simulink model "mavsim_modify"  (R2018b)
settings: Solver=ode15s  StartTime=0.0  StopTime=200  FixedStep=P.Ts  RelTol=1e-3  EnableMultiTasking=on
InitFcn:
  | aerosonde
  | param_chap7
values from neighbouring files (symbols this model uses):
  q = uu(11)    [drawVehicle.m]    (also in forceee.m; plotmavstatevariables.m = 180/pi*uu(11); plotresults.m = 180/pi*uu(11))
  r = uu(12)    [drawVehicle.m]    (also in forceee.m; plotmavstatevariables.m = 180/pi*uu(12); plotresults.m = 180/pi*uu(12))
undefined symbols (not defined in the file or in its folder): altitude_state_machine, drawVehicle, forceee, forces_moments, gps, HDBK, Light, MIL, P, plotmavstatevariables, plotresults, sensors, true_states
libraries: aerolibwind2 x2, simulink x2, simulink_extras x1, aerolibobsolete x1
settings Model: Creator=beard  LastModifiedBy=xinyizhao
settings DataIOCC: LimitDataPoints=on  SaveFormat=Array  SignalLoggingSaveFormat=ModelDataLogs
settings OptimizationCC: ExpressionDepthLimit=2147483647  InitFltsAndDblsToZero=on  LifeSpan=inf
settings DebuggingCC: UnderspecifiedInitializationDetection=Classic  MergeDetectMultiDrivingBlocksExec=none  SolverPrmCheckMsg=warning  FcnCallInpInsideContextMsg=warning  StateNameClashWarn=warning  LibraryContextMissingDiagnostic=none  SFUnexpectedBacktrackingDiag=warning  SFNoUnconditionalDefaultTransitionDiag=warning  SFExecutionAtInitializationDiag=none
settings HardwareCC: ProdBitPerPointer=32  ProdBitPerSizeT=32  ProdBitPerPtrDiffT=32  ProdLargestAtomicFloat=None  ProdIntDivRoundTo=Undefined  ProdEndianess=Unspecified  ProdWordSize=32  ProdHWDeviceType=32-bit Generic
settings ModelReferenceCC: PropagateSignalLabelsOutOfModel=off
settings SFSimCC: SimUseLocalCustomCode=off
settings RTWCC: RTWUseLocalCustomCode=off
settings CodeAppCC: StateflowObjectComments=on
settings GRTTargetCC: TargetLangStandard=C89/C90 (ANSI)  GeneratePreprocessorConditionals=Disable all  CombineOutputUpdateFcns=off  GRTInterface=on
settings ConfigComp: CovMetricSettings=dw  CovHtmlReporting=on  CovSaveCumulativeToWorkspaceVar=on  CovSaveSingleToWorkspaceVar=on  CovExternalEMLEnable=off  CovSFcnEnable=off

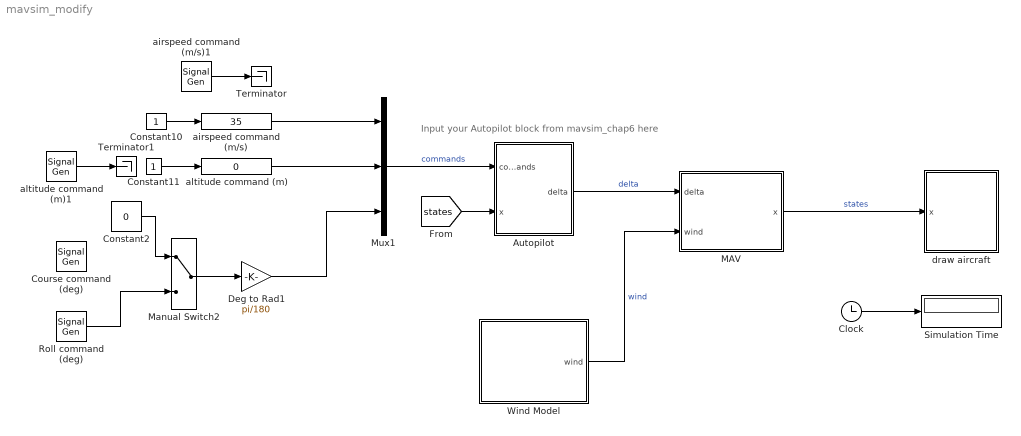
== system mavsim_modify ==
  note: Input your Autopilot block from mavsim_chap6 here
  Autopilot : Subsystem
      mask Display: image(imread('px4.png'))
  Clock : Clock
  Constant10 : Constant
  Constant11 : Constant
  Constant2 : Constant  Value=0
  Course command (deg) : SignalGenerator  WaveForm=square  Amplitude=20  Frequency=.05
  Deg to Rad1 : Gain  Gain=pi/180
  MAV : Subsystem
      mask Display: image(imread('mav.png'))
  Manual Switch2 : ManualSwitch
  Mux1 : Mux  Inputs=3
  Roll command (deg) : SignalGenerator  WaveForm=square  Amplitude=20  Frequency=.05
  Simulation Time : Display
  Terminator : Terminator
  Terminator1 : Terminator
  Wind Model : Subsystem
      mask Display: image('wind.jpg');
  airspeed command (m/s) : simulink/Math Operations/Slider Gain  gain=35  low=5  high=50
  airspeed command (m/s)1 : SignalGenerator  WaveForm=square  Amplitude=4  Frequency=.02
  altitude command (m) : simulink/Math Operations/Slider Gain  gain=0  low=0  high=500
  altitude command (m)1 : SignalGenerator  WaveForm=square  Amplitude=20  Frequency=.03
  draw aircraft : Subsystem
      mask Display: image(imread('tv.jpg'))
  wires:
  Clock/1 -> Simulation Time/1
  Wind Model/1(wind) -> MAV/2(wind)  "wind"
  MAV/1(x) -> draw aircraft/1(x)  "states"
  Autopilot/1(delta) -> MAV/1(delta)  "delta"
  Mux1/1 -> Autopilot/1(commands)  "commands"
  [states] -> Autopilot/2(x)
  Constant10/1 -> airspeed command (m/s)/1
  Deg to Rad1/1 -> Mux1/3
  airspeed command (m/s)/1 -> Mux1/1
  Constant11/1 -> altitude command (m)/1
  altitude command (m)/1 -> Mux1/2
  Manual Switch2/1 -> Deg to Rad1/1
  Roll command (deg)/1 -> Manual Switch2/2
  Constant2/1 -> Manual Switch2/1
  airspeed command (m/s)1/1 -> Terminator/1
  altitude command (m)1/1 -> Terminator1/1

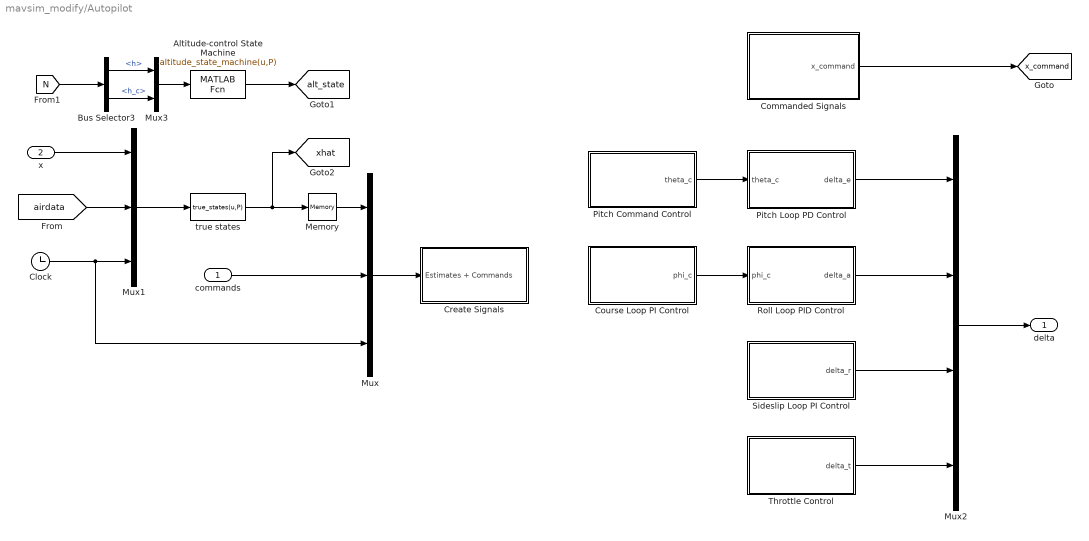
== system mavsim_modify/Autopilot ==
  commands : Inport
  x : Inport  Port=2
  Altitude-control State Machine : MATLABFcn  MATLABFcn=altitude_state_machine(u,P)  OutputDimensions=1  SampleTime=P.Ts
  Bus Selector3 : BusSelector  OutputSignals=h,h_c
  Clock : Clock
  Commanded Signals : Subsystem
  Course Loop PI Control : Subsystem
  Create Signals : Subsystem
  Memory : Memory
  Mux : Mux  Inputs=3
  Mux1 : Mux  Inputs=3
  Mux2 : Mux
  Mux3 : Mux  Inputs=2
  Pitch Command Control : Subsystem
  Pitch Loop PD Control : Subsystem
  Roll Loop PID Control : Subsystem
  Sideslip Loop PI Control : Subsystem
  Throttle Control : Subsystem
  true states : MATLABFcn  MATLABFcn=true_states(u,P)  OutputDimensions=19  SampleTime=P.Ts
  delta : Outport
  tag scope: alt_state=global, x_command=global, xhat=global
  wires:
  Clock/1 -> Mux/3, Mux1/3
  Mux2/1 -> delta/1
  commands/1 -> Mux/2
  Mux1/1 -> true states/1
  x/1 -> Mux1/1
  true states/1 -> [xhat], Memory/1
  [airdata] -> Mux1/2
  Memory/1 -> Mux/1
  Mux/1 -> Create Signals/1(Estimates + Commands)
  Pitch Loop PD Control/1(delta_e) -> Mux2/1
  Sideslip Loop PI Control/1(delta_r) -> Mux2/3
  Throttle Control/1(delta_t) -> Mux2/4
  Commanded Signals/1(x_command) -> [x_command]
  Altitude-control State Machine/1 -> [alt_state]
  [N] -> Bus Selector3/1
  Bus Selector3/1 -> Mux3/1  "<h>"
  Pitch Command Control/1(theta_c) -> Pitch Loop PD Control/1(theta_c)
  Bus Selector3/2 -> Mux3/2  "<h_c>"
  Mux3/1 -> Altitude-control State Machine/1
  Course Loop PI Control/1(phi_c) -> Roll Loop PID Control/1(phi_c)
  Roll Loop PID Control/1(delta_a) -> Mux2/2

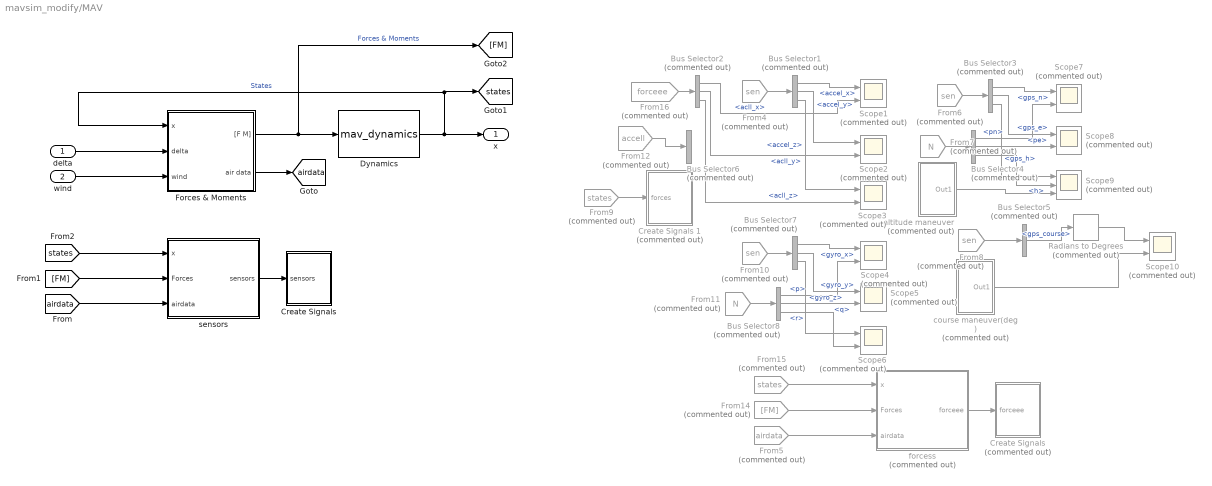
== system mavsim_modify/MAV ==
  delta : Inport
  wind : Inport  Port=2
  Bus Selector1 : BusSelector  Commented=on  OutputSignals=accel_x,accel_y,accel_z
  Bus Selector2 : BusSelector  Commented=on  OutputSignals=acll_x,acll_y,acll_z
  Bus Selector3 : BusSelector  Commented=on  OutputSignals=gps_n,gps_e,gps_h
  Bus Selector4 : BusSelector  Commented=on  OutputSignals=pn,pe,h
  Bus Selector5 : BusSelector  Commented=on  OutputSignals=gps_course
  Bus Selector6 : BusSelector  Commented=on  OutputSignals=u_dot,v_dot,w_dot
  Bus Selector7 : BusSelector  Commented=on  OutputSignals=gyro_x,gyro_y,gyro_z
  Bus Selector8 : BusSelector  Commented=on  OutputSignals=p,q,r
  Create Signals : Subsystem
  "Create Signals " : Subsystem  Commented=on
  Create Signals 1 : Subsystem  Commented=on
  Dynamics : S-Function  FunctionName=mav_dynamics  Parameters=P  SFunctionDeploymentMode=off  EnableBusSupport=off
  Forces & Moments : Subsystem
  From{4,6,8,10} (4 alike) : From  Commented=on  GotoTag=sen  TagVisibility=global
  From11 : From  Commented=on  GotoTag=N  TagVisibility=global
  From12 : From  Commented=on  GotoTag=accell  TagVisibility=global
  From14 : From  Commented=on  GotoTag=FM
  From15 : From  Commented=on  GotoTag=states  TagVisibility=global
  From16 : From  Commented=on  GotoTag=forceee  TagVisibility=global
  From5 : From  Commented=on  GotoTag=airdata  TagVisibility=global
  From7 : From  Commented=on  GotoTag=N  TagVisibility=global
  From9 : From  Commented=on  GotoTag=states  TagVisibility=global
  Radians to Degrees : simulink_extras/Transformations/Radians to Degrees  Commented=on
  Scope{1..8,10} (9 alike) : Scope  Commented=on  NumInputPorts=2
  Scope9 : Scope  Commented=on  NumInputPorts=3
  altitude maneuver : Subsystem  Commented=on
  course maneuver(deg) : Subsystem  Commented=on
  forcess : Subsystem  Commented=on
  sensors : Subsystem
  x : Outport
  tag scope: airdata=global, states=global
  wires:
  Dynamics/1 -> [states], Forces & Moments/1(x), x/1  "States"
  Forces & Moments/1("[F M]") -> [FM], Dynamics/1  "Forces & Moments"
  Forces & Moments/2(air data) -> [airdata]
  delta/1 -> Forces & Moments/2(delta)
  wind/1 -> Forces & Moments/3(wind)
  [airdata] -> sensors/3(airdata)
  [FM] -> sensors/2(Forces)
  [states] -> sensors/1(x)
  sensors/1(sensors) -> Create Signals/1(sensors)
  Bus Selector1/3 -> Scope3/1  "<accel_z>"
  From11/1 -> Bus Selector8/1
  From10/1 -> Bus Selector7/1
  Bus Selector7/2 -> Scope5/1  "<gyro_y>"
  From4/1 -> Bus Selector1/1
  Radians to Degrees/1 -> Scope10/1
  Bus Selector4/3 -> Scope9/2  "<h>"
  Bus Selector5/1 -> Radians to Degrees/1  "<gps_course>"
  From6/1 -> Bus Selector3/1
  Bus Selector7/1 -> Scope4/1  "<gyro_x>"
  Bus Selector8/1 -> Scope4/2  "<p>"
  Bus Selector1/1 -> Scope1/1  "<accel_x>"
  Bus Selector1/2 -> Scope2/1  "<accel_y>"
  Bus Selector3/2 -> Scope8/1  "<gps_e>"
  Bus Selector4/1 -> Scope7/2  "<pn>"
  Bus Selector8/2 -> Scope5/2  "<q>"
  Bus Selector3/3 -> Scope9/1  "<gps_h>"
  Bus Selector8/3 -> Scope6/2  "<r>"
  Bus Selector7/3 -> Scope6/1  "<gyro_z>"
  Bus Selector4/2 -> Scope8/2  "<pe>"
  Bus Selector3/1 -> Scope7/1  "<gps_n>"
  From7/1 -> Bus Selector4/1
  course maneuver(deg)/1(Out1) -> Scope10/2
  From8/1 -> Bus Selector5/1
  From5/1 -> forcess/3(airdata)
  forcess/1(forceee) -> "Create Signals "/1(forceee)
  From15/1 -> forcess/1(x)
  From14/1 -> forcess/2(Forces)
  From16/1 -> Bus Selector2/1
  From9/1 -> Create Signals 1/1(forces)
  From12/1 -> Bus Selector6/1
  Bus Selector2/1 -> Scope1/2  "<acll_x>"
  Bus Selector2/2 -> Scope2/2  "<acll_y>"
  Bus Selector2/3 -> Scope3/2  "<acll_z>"
  altitude maneuver/1(Out1) -> Scope9/3

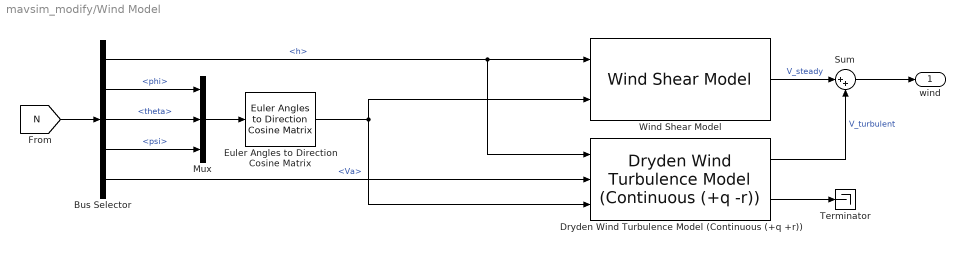
== system mavsim_modify/Wind Model ==
  Bus Selector : BusSelector  OutputSignals=h,phi,theta,psi,Va
  Dryden Wind Turbulence Model (Continuous (+q +r)) : aerolibwind2/Dryden Wind Turbulence Model  (Continuous (+q -r))  units=Metric (MKS)  spec=MIL-HDBK-1797  model=Continuous Dryden (+q +r)  W20=P.w_mag  Wdeg=P.w_dir  TurbProb=10^-2 - Light  L_high=533.4  Wingspan=P.b  ts=P.Ts  Seed=[23341 23342 0 23344]  T_on=off
      settings: SourceProductName=Aerospace Blockset
  Euler Angles to Direction Cosine Matrix : aerolibobsolete/Euler Angles to  Direction Cosine Matrix
      settings: SourceProductName=Aerospace Blockset  SourceProductBaseCode=AE
  Mux : Mux  Inputs=3
  Sum : Sum  Inputs=|++
  Terminator : Terminator
  Wind Shear Model : aerolibwind2/Wind Shear Model  units=Metric (MKS)  phase=Category C - Terminal Flight Phase  W_20=P.w_mag  Wdeg=P.w_dir
      settings: SourceProductName=Aerospace Blockset
  wind : Outport
  wires:
  Dryden Wind Turbulence Model (Continuous (+q +r))/2 -> Terminator/1
  Euler Angles to Direction Cosine Matrix/1 -> Dryden Wind Turbulence Model (Continuous (+q +r))/3, Wind Shear Model/2
  Wind Shear Model/1 -> Sum/1  "V_steady"
  Bus Selector/5 -> Dryden Wind Turbulence Model (Continuous (+q +r))/2  "<Va>"
  Bus Selector/1 -> Dryden Wind Turbulence Model (Continuous (+q +r))/1, Wind Shear Model/1  "<h>"
  Dryden Wind Turbulence Model (Continuous (+q +r))/1 -> Sum/2  "V_turbulent"
  Bus Selector/2 -> Mux/1  "<phi>"
  Bus Selector/3 -> Mux/2  "<theta>"
  Bus Selector/4 -> Mux/3  "<psi>"
  Mux/1 -> Euler Angles to Direction Cosine Matrix/1
  Sum/1 -> wind/1
  [N] -> Bus Selector/1

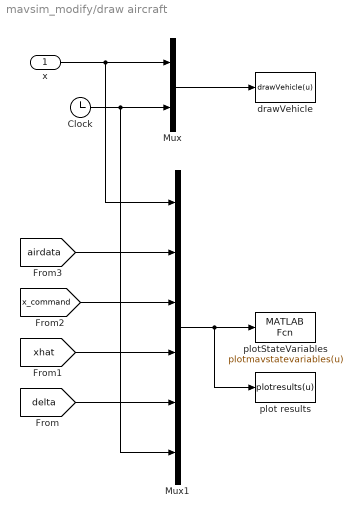
== system mavsim_modify/draw aircraft ==
  x : Inport
  Clock : Clock
  Mux : Mux  Inputs=2
  Mux1 : Mux  Inputs=6
  drawVehicle : MATLABFcn  MATLABFcn=drawVehicle(u)  OutputDimensions=0  SampleTime=0.1
  plot results : MATLABFcn  MATLABFcn=plotresults(u)  OutputDimensions=0  SampleTime=0.1
  plotStateVariables : MATLABFcn  MATLABFcn=plotmavstatevariables(u)  OutputDimensions=0  SampleTime=0.1
  wires:
  Mux/1 -> drawVehicle/1
  x/1 -> Mux/1, Mux1/1
  Clock/1 -> Mux/2, Mux1/6
  [xhat] -> Mux1/4
  [x_command] -> Mux1/3
  [delta] -> Mux1/5
  [airdata] -> Mux1/2
  Mux1/1 -> plot results/1, plotStateVariables/1

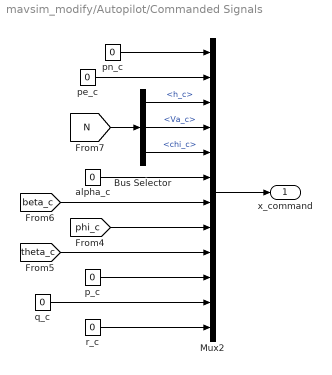
== system mavsim_modify/Autopilot/Commanded Signals ==
  Bus Selector : BusSelector  OutputSignals=h_c,Va_c,chi_c
  Mux2 : Mux  Inputs=12
  alpha_c : Constant  Value=0
  p_c : Constant  Value=0
  pe_c : Constant  Value=0
  pn_c : Constant  Value=0
  q_c : Constant  Value=0
  r_c : Constant  Value=0
  x_command : Outport
  wires:
  Bus Selector/1 -> Mux2/3  "<h_c>"
  pe_c/1 -> Mux2/2
  p_c/1 -> Mux2/10
  Mux2/1 -> x_command/1
  alpha_c/1 -> Mux2/6
  pn_c/1 -> Mux2/1
  Bus Selector/2 -> Mux2/4  "<Va_c>"
  [beta_c] -> Mux2/7
  Bus Selector/3 -> Mux2/5  "<chi_c>"
  q_c/1 -> Mux2/11
  [N] -> Bus Selector/1
  r_c/1 -> Mux2/12
  [phi_c] -> Mux2/8
  [theta_c] -> Mux2/9

== system mavsim_modify/Autopilot/Course Loop PI Control ==
  Bus Selector3 : BusSelector  OutputSignals=chi_c,chi
  Gain : Gain  Gain=P.course_kp
  Roll Saturation : Saturate  UpperLimit=P.phi_max  LowerLimit=-1*P.phi_max
  Sum : Sum
  Sum4 : Sum  Inputs=|+-
  course_ki : TransferFcn  Numerator=[P.course_ki]  Denominator=[1 0]
  phi_c : Outport
  wires:
  [N] -> Bus Selector3/1
  Bus Selector3/2 -> Sum4/2  "<chi>"
  Bus Selector3/1 -> Sum4/1  "<chi_c>"
  Roll Saturation/1 -> phi_c/1
  Sum4/1 -> Gain/1, course_ki/1  "course_e"
  Gain/1 -> Sum/2
  course_ki/1 -> Sum/1
  Sum/1 -> Roll Saturation/1

== system mavsim_modify/Autopilot/Create Signals ==
  Estimates + Commands : Inport
  Bus Creator : BusCreator  Inputs=23
  Demux1 : Demux  Outputs=23
  tag scope: N=global
  wires:
  Demux1/14 -> Bus Creator/14  "wn"
  Demux1/4 -> Bus Creator/4  "Va"
  Demux1/2 -> Bus Creator/2  "pe"
  Demux1/21 -> Bus Creator/21  "h_c"
  Demux1/15 -> Bus Creator/15  "we"
  Demux1/13 -> Bus Creator/13  "Vg"
  Demux1/18 -> Bus Creator/18  "by"
  Estimates + Commands/1 -> Demux1/1
  Demux1/9 -> Bus Creator/9  "chi"
  Demux1/17 -> Bus Creator/17  "bx"
  Demux1/16 -> Bus Creator/16  "psi"
  Demux1/20 -> Bus Creator/20  "Va_c"
  Demux1/19 -> Bus Creator/19  "bz"
  Demux1/5 -> Bus Creator/5  "alpha"
  Demux1/23 -> Bus Creator/23  "t"
  Demux1/10 -> Bus Creator/10  "p"
  Demux1/12 -> Bus Creator/12  "r"
  Demux1/11 -> Bus Creator/11  "q"
  Bus Creator/1 -> [N]
  Demux1/22 -> Bus Creator/22  "chi_c"
  Demux1/3 -> Bus Creator/3  "h"
  Demux1/8 -> Bus Creator/8  "theta"
  Demux1/6 -> Bus Creator/6  "beta"
  Demux1/7 -> Bus Creator/7  "phi"
  Demux1/1 -> Bus Creator/1  "pn"

== system mavsim_modify/Autopilot/Pitch Command Control ==
  Airspeed Hold Using Pitch Loop PI Control : Subsystem
  "Airspeed Hold Using Pitch Loop PI Control " : Subsystem
  Altitude Hold Using Pitch Loop PI Control : Subsystem
  Constant : Constant  Value=P.theta_max
  Multiport Switch : MultiPortSwitch  Inputs=4  DataPortIndices={10,2,3}  DiagnosticForDefault=None
  Pitch Saturation : Saturate  UpperLimit=P.theta_max  LowerLimit=-1*P.theta_max
  theta_c : Outport
  wires:
  Altitude Hold Using Pitch Loop PI Control/1(theta_c) -> Multiport Switch/4  "Altitude Hold Zone"
  Airspeed Hold Using Pitch Loop PI Control/1(theta_c) -> Multiport Switch/3  "Climb Zone"
  [alt_state] -> Multiport Switch/1  "Altitude-control State Variable"
  Constant/1 -> Multiport Switch/2  "Take-off Zone"
  "Airspeed Hold Using Pitch Loop PI Control "/1(theta_c) -> Multiport Switch/5  "Descend Zone"
  Multiport Switch/1 -> Pitch Saturation/1
  Pitch Saturation/1 -> theta_c/1

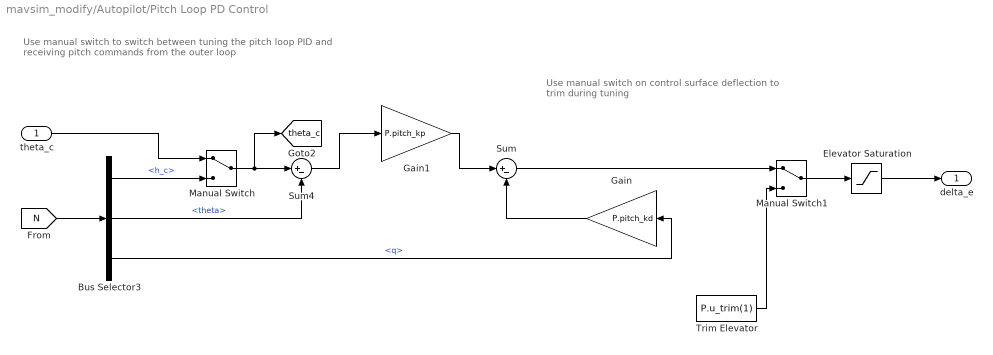
== system mavsim_modify/Autopilot/Pitch Loop PD Control ==
  note: Use manual switch to switch between tuning the pitch loop PID and
      | receiving pitch commands from the outer loop
  note: Use manual switch on control surface deflection
      | to trim during tuning
  theta_c : Inport
  Bus Selector3 : BusSelector  OutputSignals=h_c,theta,q
  Elevator Saturation : Saturate  UpperLimit=P.delta_e_max  LowerLimit=-1*P.delta_e_max
  Gain : Gain  Gain=P.pitch_kd
  Gain1 : Gain  Gain=P.pitch_kp
  Manual Switch : ManualSwitch
  Manual Switch1 : ManualSwitch
  Sum : Sum  Inputs=|+-
  Sum4 : Sum  Inputs=|+-
  Trim Elevator : Constant  Value=P.u_trim(1)
  delta_e : Outport
  tag scope: theta_c=global
  wires:
  Manual Switch/1 -> [theta_c], Sum4/1
  theta_c/1 -> Manual Switch/1
  [N] -> Bus Selector3/1
  Bus Selector3/2 -> Sum4/2  "<theta>"
  Bus Selector3/1 -> Manual Switch/2  "<h_c>"
  Trim Elevator/1 -> Manual Switch1/2
  Manual Switch1/1 -> Elevator Saturation/1
  Sum4/1 -> Gain1/1
  Bus Selector3/3 -> Gain/1  "<q>"
  Gain1/1 -> Sum/1
  Gain/1 -> Sum/2
  Sum/1 -> Manual Switch1/1
  Elevator Saturation/1 -> delta_e/1

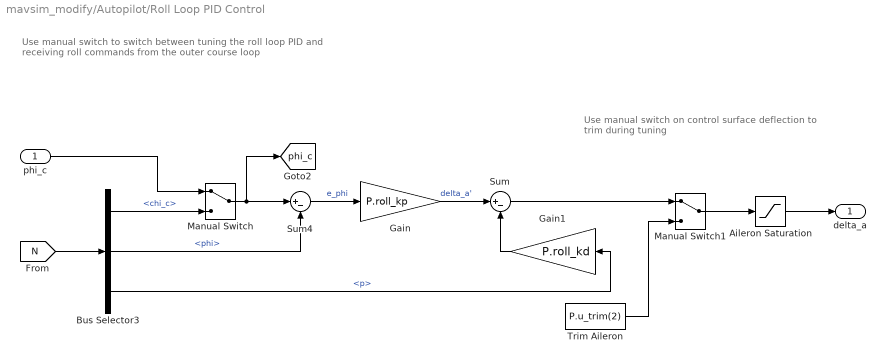
== system mavsim_modify/Autopilot/Roll Loop PID Control ==
  note: Use manual switch on control surface deflection
      | to trim during tuning
  note: Use manual switch to switch between tuning the roll loop PID and
      | receiving roll commands from the outer course loop
  phi_c : Inport
  Aileron Saturation : Saturate  UpperLimit=P.delta_a_max  LowerLimit=-1*P.delta_a_max
  Bus Selector3 : BusSelector  OutputSignals=chi_c,phi,p
  Gain : Gain  Gain=P.roll_kp
  Gain1 : Gain  Gain=P.roll_kd
  Manual Switch : ManualSwitch
  Manual Switch1 : ManualSwitch
  Sum : Sum  Inputs=|+-
  Sum4 : Sum  Inputs=|+-
  Trim Aileron : Constant  Value=P.u_trim(2)
  delta_a : Outport
  tag scope: phi_c=global
  wires:
  Bus Selector3/1 -> Manual Switch/2  "<chi_c>"
  Bus Selector3/2 -> Sum4/2  "<phi>"
  [N] -> Bus Selector3/1
  phi_c/1 -> Manual Switch/1
  Manual Switch/1 -> [phi_c], Sum4/1
  Aileron Saturation/1 -> delta_a/1
  Trim Aileron/1 -> Manual Switch1/2
  Manual Switch1/1 -> Aileron Saturation/1
  Sum4/1 -> Gain/1  "e_phi"
  Gain/1 -> Sum/1  "delta_a'"
  Gain1/1 -> Sum/2
  Sum/1 -> Manual Switch1/1
  Bus Selector3/3 -> Gain1/1  "<p>"

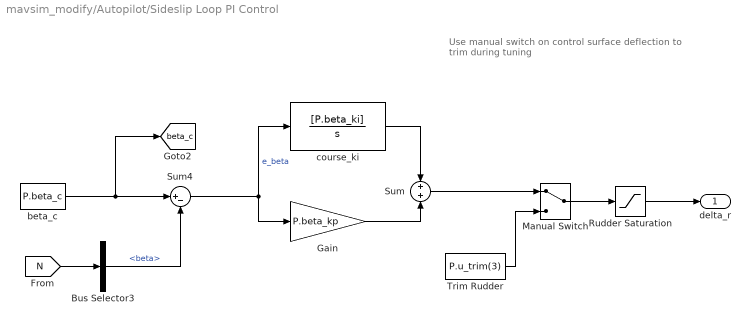
== system mavsim_modify/Autopilot/Sideslip Loop PI Control ==
  note: Use manual switch on control surface deflection
      | to trim during tuning
  Bus Selector3 : BusSelector  OutputSignals=beta
  Gain : Gain  Gain=P.beta_kp
  Manual Switch : ManualSwitch
  Rudder Saturation : Saturate  UpperLimit=P.delta_r_max  LowerLimit=-1*P.delta_r_max
  Sum : Sum
  Sum4 : Sum  Inputs=|+-
  Trim Rudder : Constant  Value=P.u_trim(3)
  beta_c : Constant  Value=P.beta_c
  course_ki : TransferFcn  Numerator=[P.beta_ki]  Denominator=[1 0]
  delta_r : Outport
  tag scope: beta_c=global
  wires:
  [N] -> Bus Selector3/1
  Bus Selector3/1 -> Sum4/2  "<beta>"
  beta_c/1 -> [beta_c], Sum4/1
  Manual Switch/1 -> Rudder Saturation/1
  Trim Rudder/1 -> Manual Switch/2
  Rudder Saturation/1 -> delta_r/1
  Sum4/1 -> Gain/1, course_ki/1  "e_beta"
  course_ki/1 -> Sum/1
  Sum/1 -> Manual Switch/1
  Gain/1 -> Sum/2

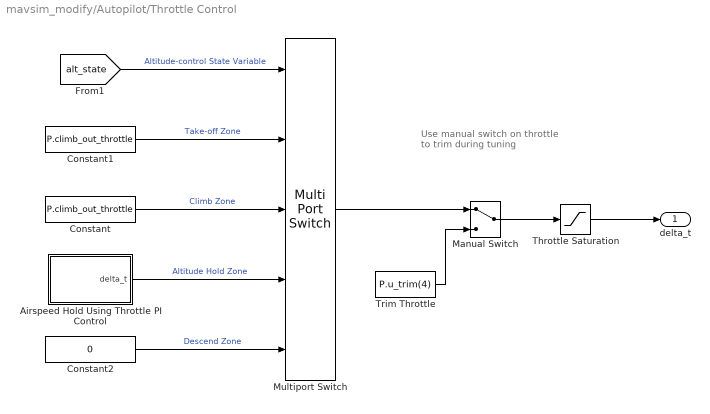
== system mavsim_modify/Autopilot/Throttle Control ==
  note: Use manual switch on throttle
      | to trim during tuning
  Airspeed Hold Using Throttle PI Control : Subsystem
  Constant : Constant  Value=P.climb_out_throttle
  Constant1 : Constant  Value=P.climb_out_throttle
  Constant2 : Constant  Value=0
  Manual Switch : ManualSwitch
  Multiport Switch : MultiPortSwitch  Inputs=4  DataPortIndices={10,2,3}  DiagnosticForDefault=None
  Throttle Saturation : Saturate  UpperLimit=P.throttle_max  LowerLimit=0
  Trim Throttle : Constant  Value=P.u_trim(4)
  delta_t : Outport
  wires:
  Multiport Switch/1 -> Manual Switch/1
  Airspeed Hold Using Throttle PI Control/1(delta_t) -> Multiport Switch/4  "Altitude Hold Zone"
  [alt_state] -> Multiport Switch/1  "Altitude-control State Variable"
  Constant/1 -> Multiport Switch/3  "Climb Zone"
  Constant1/1 -> Multiport Switch/2  "Take-off Zone"
  Constant2/1 -> Multiport Switch/5  "Descend Zone"
  Throttle Saturation/1 -> delta_t/1
  Trim Throttle/1 -> Manual Switch/2
  Manual Switch/1 -> Throttle Saturation/1

== system mavsim_modify/MAV/Create Signals ==
  sensors : Inport
  Bus Creator : BusCreator  Inputs=13
  Demux1 : Demux  Outputs=13
  tag scope: sen=global
  wires:
  sensors/1 -> Demux1/1
  Bus Creator/1 -> [sen]
  Demux1/1 -> Bus Creator/1  "gyro_x"
  Demux1/2 -> Bus Creator/2  "gyro_y"
  Demux1/3 -> Bus Creator/3  "gyro_z"
  Demux1/4 -> Bus Creator/4  "accel_x"
  Demux1/5 -> Bus Creator/5  "accel_y"
  Demux1/6 -> Bus Creator/6  "accel_z"
  Demux1/7 -> Bus Creator/7  "static_pres"
  Demux1/8 -> Bus Creator/8  "diff_pres"
  Demux1/9 -> Bus Creator/9  "gps_n"
  Demux1/10 -> Bus Creator/10  "gps_e"
  Demux1/11 -> Bus Creator/11  "gps_h"
  Demux1/12 -> Bus Creator/12  "gps_Vg"
  Demux1/13 -> Bus Creator/13  "gps_course"

== system mavsim_modify/MAV/Create Signals  ==
  forceee : Inport
  Bus Creator : BusCreator  Inputs=3
  Demux1 : Demux  Outputs=3
  tag scope: forceee=global
  wires:
  forceee/1 -> Demux1/1
  Bus Creator/1 -> [forceee]
  Demux1/1 -> Bus Creator/1  "acll_x"
  Demux1/2 -> Bus Creator/2  "acll_y"
  Demux1/3 -> Bus Creator/3  "acll_z"

== system mavsim_modify/MAV/Create Signals 1 ==
  forces : Inport
  Bus Creator : BusCreator  Inputs=12
  Demux1 : Demux  Outputs=12
  tag scope: accell=global
  wires:
  forces/1 -> Demux1/1
  Bus Creator/1 -> [accell]
  Demux1/1 -> Bus Creator/1
  Demux1/2 -> Bus Creator/2
  Demux1/3 -> Bus Creator/3
  Demux1/4 -> Bus Creator/4  "u_dot"
  Demux1/5 -> Bus Creator/5  "v_dot"
  Demux1/6 -> Bus Creator/6  "w_dot"
  Demux1/7 -> Bus Creator/7
  Demux1/8 -> Bus Creator/8
  Demux1/9 -> Bus Creator/9
  Demux1/10 -> Bus Creator/10
  Demux1/11 -> Bus Creator/11
  Demux1/12 -> Bus Creator/12

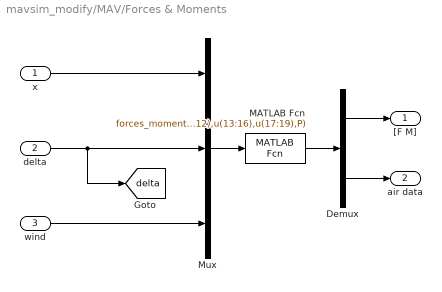
== system mavsim_modify/MAV/Forces & Moments ==
  x : Inport
  delta : Inport  Port=2
  wind : Inport  Port=3
  Demux : Demux  Outputs=[6;6]
  MATLAB Fcn : MATLABFcn  MATLABFcn=forces_moments(u(1:12),u(13:16),u(17:19),P)  OutputDimensions=12
  Mux : Mux  Inputs=3
  "[F M]" : Outport
  air data : Outport  Port=2
  tag scope: delta=global
  wires:
  Demux/2 -> air data/1
  Mux/1 -> MATLAB Fcn/1
  Demux/1 -> "[F M]"/1
  MATLAB Fcn/1 -> Demux/1
  wind/1 -> Mux/3
  delta/1 -> Mux/2, [delta]
  x/1 -> Mux/1

== system mavsim_modify/MAV/altitude maneuver ==
  Add : Sum  Inputs=++++
  Step : Step  Time=0  After=100  SampleTime=0
  Step1 : Step  Time=20  After=20  SampleTime=0
  Step2 : Step  Time=50  After=-40  SampleTime=0
  Step3 : Step  Time=80  After=20  SampleTime=0
  Out1 : Outport
  wires:
  Step2/1 -> Add/3
  Step3/1 -> Add/4
  Step/1 -> Add/1
  Add/1 -> Out1/1
  Step1/1 -> Add/2

== system mavsim_modify/MAV/course maneuver(deg) ==
  Add1 : Sum  Inputs=+++
  Step5 : Step  Time=5  After=30  SampleTime=0
  Step6 : Step  Time=15  After=-60  SampleTime=0
  Step7 : Step  Time=30  After=30  SampleTime=0
  Out1 : Outport
  wires:
  Add1/1 -> Out1/1
  Step5/1 -> Add1/2
  Step6/1 -> Add1/3
  Step7/1 -> Add1/1

== system mavsim_modify/MAV/forcess ==
  x : Inport
  Forces : Inport  Port=2
  airdata : Inport  Port=3
  Clock : Clock
  Mux2 : Mux
  "forceee " : MATLABFcn  MATLABFcn=forceee(u,P)  OutputDimensions=3  SampleTime=P.Ts
  forceee : Outport
  wires:
  Mux2/1 -> "forceee "/1
  Forces/1 -> Mux2/2
  airdata/1 -> Mux2/3
  "forceee "/1 -> forceee/1
  x/1 -> Mux2/1
  Clock/1 -> Mux2/4

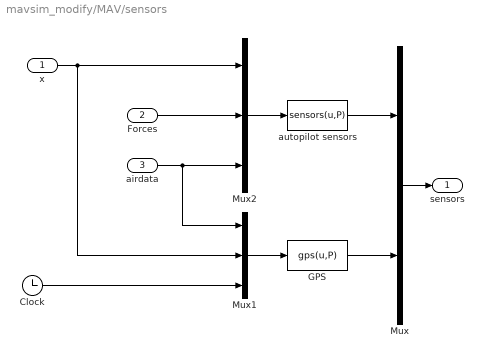
== system mavsim_modify/MAV/sensors ==
  x : Inport
  Forces : Inport  Port=2
  airdata : Inport  Port=3
  Clock : Clock
  GPS : MATLABFcn  MATLABFcn=gps(u,P)  OutputDimensions=5  SampleTime=P.Ts_gps
  Mux : Mux  Inputs=2
  Mux1 : Mux  Inputs=3
  Mux2 : Mux  Inputs=3
  autopilot sensors : MATLABFcn  MATLABFcn=sensors(u,P)  OutputDimensions=8  SampleTime=P.Ts
  sensors : Outport
  wires:
  autopilot sensors/1 -> Mux/1
  GPS/1 -> Mux/2
  Mux1/1 -> GPS/1
  Clock/1 -> Mux1/3
  Mux2/1 -> autopilot sensors/1
  Forces/1 -> Mux2/2
  airdata/1 -> Mux2/3, Mux1/1
  Mux/1 -> sensors/1
  x/1 -> Mux2/1, Mux1/2

== system mavsim_modify/Autopilot/Pitch Command Control/Airspeed Hold Using Pitch Loop PI Control ==
  Altitude State Check : Subsystem
  Bus Selector3 : BusSelector  OutputSignals=Va_c,Va
  Gain : Gain  Gain=P.airspeed_pitch_kp
  Sum : Sum
  Sum4 : Sum  Inputs=|+-
  ki : TransferFcn  Numerator=[P.airspeed_pitch_ki]  Denominator=[1 0]
  theta_c : Outport
  wires:
  [N] -> Bus Selector3/1
  Bus Selector3/2 -> Sum4/2  "<Va>"
  Bus Selector3/1 -> Sum4/1  "<Va_c>"
  Sum4/1 -> Altitude State Check/1(err_in)
  Altitude State Check/1(err_out) -> Gain/1, ki/1
  ki/1 -> Sum/1
  Gain/1 -> Sum/2
  Sum/1 -> theta_c/1

== system mavsim_modify/Autopilot/Pitch Command Control/Airspeed Hold Using Pitch Loop PI Control  ==
  Altitude State Check : Subsystem
  Bus Selector3 : BusSelector  OutputSignals=Va_c,Va
  Gain : Gain  Gain=P.airspeed_pitch_kp
  Sum : Sum
  Sum4 : Sum  Inputs=|+-
  course_ki : TransferFcn  Numerator=[P.airspeed_pitch_ki]  Denominator=[1 0]
  theta_c : Outport
  wires:
  Sum4/1 -> Altitude State Check/1(err_in)
  Bus Selector3/1 -> Sum4/1  "<Va_c>"
  Sum/1 -> theta_c/1
  Bus Selector3/2 -> Sum4/2  "<Va>"
  [N] -> Bus Selector3/1
  Altitude State Check/1(err_out) -> Gain/1, course_ki/1
  course_ki/1 -> Sum/1
  Gain/1 -> Sum/2

== system mavsim_modify/Autopilot/Pitch Command Control/Altitude Hold Using Pitch Loop PI Control ==
  Altitude State Check : Subsystem
  Bus Selector3 : BusSelector  OutputSignals=h_c,h
  Gain : Gain  Gain=P.altitude_kp
  Sum : Sum
  Sum4 : Sum  Inputs=|+-
  course_ki : TransferFcn  Numerator=[P.altitude_ki]  Denominator=[1 0]
  theta_c : Outport
  wires:
  Sum4/1 -> Altitude State Check/1(err_in)
  Bus Selector3/1 -> Sum4/1  "<h_c>"
  Sum/1 -> theta_c/1
  Bus Selector3/2 -> Sum4/2  "<h>"
  [N] -> Bus Selector3/1
  Altitude State Check/1(err_out) -> Gain/1, course_ki/1
  course_ki/1 -> Sum/1
  Gain/1 -> Sum/2

== system mavsim_modify/Autopilot/Throttle Control/Airspeed Hold Using Throttle PI Control ==
  Altitude State Check : Subsystem
  Bus Selector3 : BusSelector  OutputSignals=Va_c,Va
  Sum : Sum  Inputs=|++
  Sum4 : Sum  Inputs=|+-
  course_ki : TransferFcn  Numerator=[P.airspeed_throttle_ki]  Denominator=[1 0]
  course_kp : TransferFcn  Numerator=[P.airspeed_throttle_kp]  Denominator=[0 1]
  delta_t : Outport
  wires:
  Bus Selector3/2 -> Sum4/2  "<Va>"
  [N] -> Bus Selector3/1
  Bus Selector3/1 -> Sum4/1  "<Va_c>"
  Sum4/1 -> Altitude State Check/1(err_in)
  Altitude State Check/1(err_out) -> course_kp/1, course_ki/1  "e_beta"
  Sum/1 -> delta_t/1
  course_kp/1 -> Sum/2
  course_ki/1 -> Sum/1

== system mavsim_modify/Autopilot/Pitch Command Control/Airspeed Hold Using Pitch Loop PI Control/Altitude State Check ==
  err_in : Inport
  Climb Zone : Constant  Value=2
  Product : Product
  Relational Operator : RelationalOperator  Operator===  OutDataTypeStr=boolean  RndMeth=Simplest
  err_out : Outport
  wires:
  err_in/1 -> Product/2
  Relational Operator/1 -> Product/1
  Product/1 -> err_out/1
  [alt_state] -> Relational Operator/1
  Climb Zone/1 -> Relational Operator/2

== system mavsim_modify/Autopilot/Pitch Command Control/Airspeed Hold Using Pitch Loop PI Control /Altitude State Check ==
  err_in : Inport
  Descend Zone : Constant  Value=4
  Product : Product
  Relational Operator : RelationalOperator  Operator===  OutDataTypeStr=boolean  RndMeth=Simplest
  err_out : Outport
  wires:
  err_in/1 -> Product/2
  Relational Operator/1 -> Product/1
  Product/1 -> err_out/1
  [alt_state] -> Relational Operator/1
  Descend Zone/1 -> Relational Operator/2

== system mavsim_modify/Autopilot/Pitch Command Control/Altitude Hold Using Pitch Loop PI Control/Altitude State Check ==
  err_in : Inport
  Alt Hold Zone : Constant  Value=3
  Product : Product
  Relational Operator : RelationalOperator  Operator===  OutDataTypeStr=boolean  RndMeth=Simplest
  err_out : Outport
  wires:
  err_in/1 -> Product/2
  Relational Operator/1 -> Product/1
  Product/1 -> err_out/1
  [alt_state] -> Relational Operator/1
  Alt Hold Zone/1 -> Relational Operator/2

== system mavsim_modify/Autopilot/Throttle Control/Airspeed Hold Using Throttle PI Control/Altitude State Check ==
  err_in : Inport
  Alt Hold Zone : Constant  Value=3
  Product : Product
  Relational Operator : RelationalOperator  Operator===  OutDataTypeStr=boolean  RndMeth=Simplest
  err_out : Outport
  wires:
  err_in/1 -> Product/2
  Relational Operator/1 -> Product/1
  Product/1 -> err_out/1
  [alt_state] -> Relational Operator/1
  Alt Hold Zone/1 -> Relational Operator/2
